simulink library "INT_RailP_DDsync"  (R2016b)
settings: Solver=VariableStepAuto  StartTime=0.0  StopTime=10.0  RelTol=1e-3
settings Model: Creator=lenovo  LastModifiedBy=lenovo

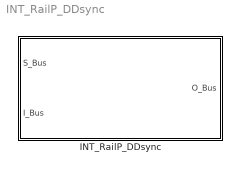
== system INT_RailP_DDsync ==
  INT_RailP_DDsync : Subsystem

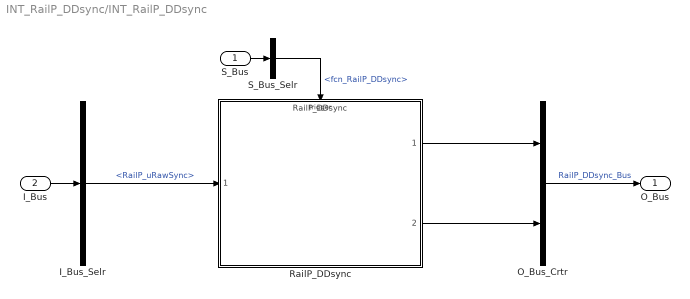
== system INT_RailP_DDsync/INT_RailP_DDsync ==
  S_Bus : Inport
  I_Bus : Inport  Port=2
  I_Bus_Selr : BusSelector  OutputSignals=RailP_uRawSync
  O_Bus_Crtr : BusCreator  Inputs=2
  RailP_DDsync : ModelReference  ModelNameDialog=RailP_DDsync  SimulationMode=Normal  ModelReferenceVersion=1.3  TriggerPortName=function  TriggerPortTriggerType=function-call  TriggerPortStatesWhenEnabling=held
  S_Bus_Selr : BusSelector  OutputSignals=fcn_RailP_DDsync
  O_Bus : Outport
  wires:
  S_Bus_Selr/1 -> RailP_DDsync/Trigger  "<fcn_RailP_DDsync>"
  S_Bus/1 -> S_Bus_Selr/1
  I_Bus/1 -> I_Bus_Selr/1
  I_Bus_Selr/1 -> RailP_DDsync/1  "<RailP_uRawSync>"
  O_Bus_Crtr/1 -> O_Bus/1  "RailP_DDsync_Bus"
  RailP_DDsync/1 -> O_Bus_Crtr/1
  RailP_DDsync/2 -> O_Bus_Crtr/2
